simulink model "simulink_test"  (R2023b)
settings: Solver=ode15s  StartTime=0.0  StopTime=10.0  RelTol=1e-3
values from neighbouring files (symbols this model uses):
  N_B = 1    [class_test2D.m]    (also in class_test3D.m; class_test_rigid.m = n; test_plot.m; test_volumetric.m)
  q_test = 1    [class_test2D.m]    (also in class_test3D.m = 1*[1; -1; 0.2]; class_test_rigid.m; test_plot.m = q_lb + (q_ub-q_lb).*rand(sr.n,1); test_volumetric.m = [1; -0.1; 0])
  r1 = BodyTree(J1, B1)    [class_test_rigid.m]    (also in methods_test.m)
libraries: SoftRobotics x1
settings Model: Creator=pietro  LastModifiedBy=pietro

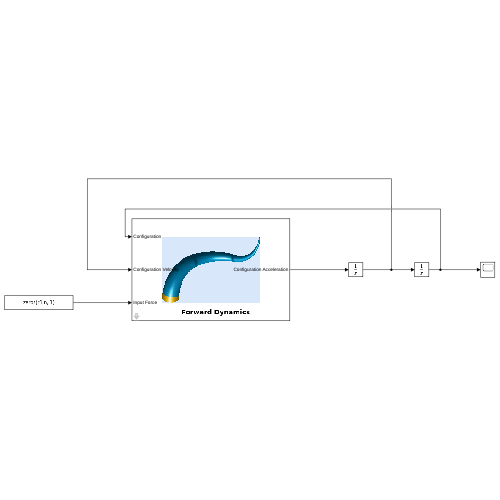
[thumbnail: Simulink's stored preview of the top-level diagram]
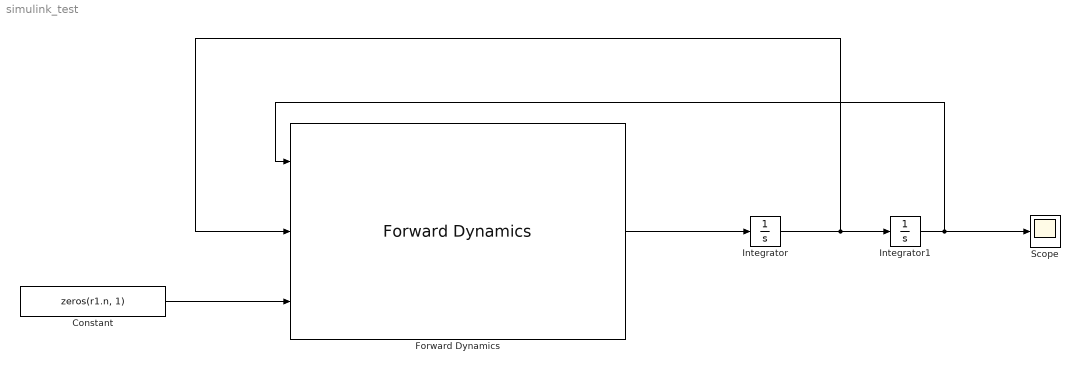
== system simulink_test ==
  Constant : Constant  Value=zeros(r1.n, 1)
  Forward Dynamics : SoftRobotics/Forward Dynamics  RobotModel=r1  SimulateUsing=Code generation
      settings: SourceProductName=Soft Robotics Toolbox
  Integrator : Integrator
  Integrator1 : Integrator  InitialCondition=repmat(q_test, N_B, 1)
  Scope : Scope
  wires:
  Forward Dynamics/1 -> Integrator/1
  Integrator/1 -> Forward Dynamics/2, Integrator1/1
  Constant/1 -> Forward Dynamics/3
  Integrator1/1 -> Forward Dynamics/1, Scope/1
